simulink model "SensingHealthCheckBlock"  (R2023a)
settings: Solver=VariableStepAuto  StartTime=0.0  StopTime=10.0  RelTol=1e-3
settings Model: Creator=aan18022  LastModifiedBy=aan18022

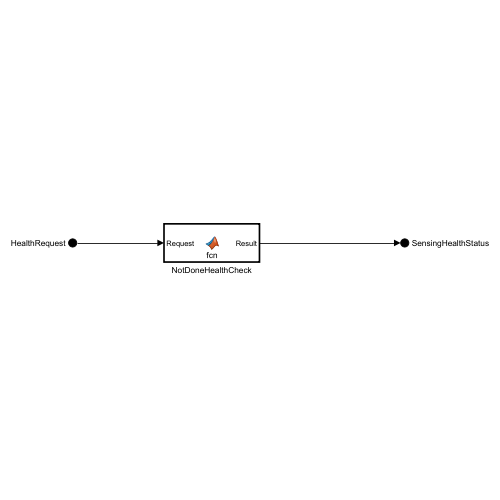
[thumbnail: Simulink's stored preview of the top-level diagram]
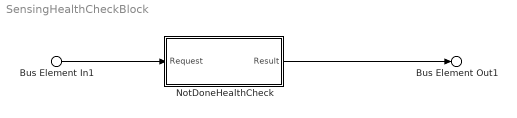
== system SensingHealthCheckBlock ==
  Bus Element In1 : Inport  PortName=HealthRequest
  NotDoneHealthCheck : MATLAB Function  TreatAsAtomicUnit=on
  Bus Element Out1 : Outport  PortName=SensingHealthStatus
  wires:
  Bus Element In1/1 -> NotDoneHealthCheck/1(Request)
  NotDoneHealthCheck/1(Result) -> Bus Element Out1/1

== matlab function SensingHealthCheckBlock/NotDoneHealthCheck ==
  data: Request input; Result output
function Result = fcn(Request)

if Request == 1
    Result = 1;
else
    Result = 0;
end
